simulink model "dynamic_resistance_charging"  (R2023a)
settings: Solver=VariableStepAuto  StartTime=0.0  StopTime=300  FixedStep=5e-6  RelTol=1e-3
undefined symbols (not defined in the file): Ion, Lithium
libraries: spsSeriesRLCBranchLib x8, spsMosfetLib x5, spsCurrentMeasurementLib x4, spsBatteryLib x3, spsDCVoltageSourceLib x1, spsGroundLib x1, sps_lib x1
settings Model: SimulationMode=accelerator  Creator=91620  LastModifiedBy=91620

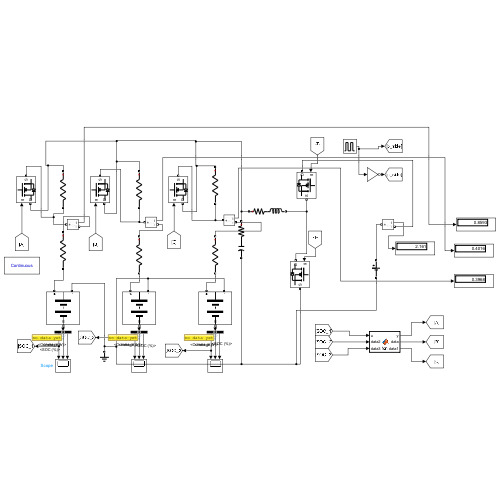
[thumbnail: Simulink's stored preview of the top-level diagram]
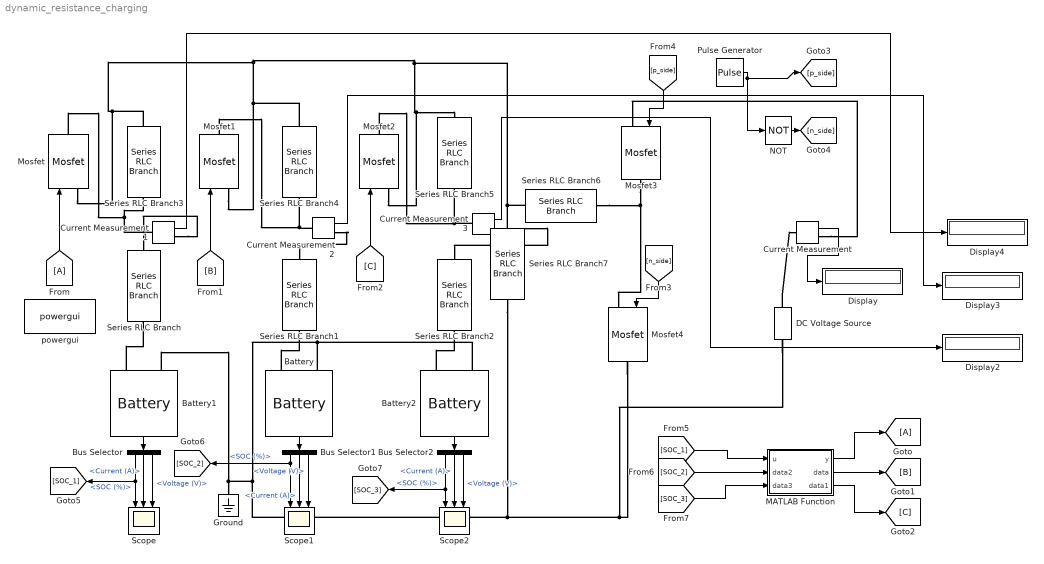
== system dynamic_resistance_charging ==
  Battery : spsBatteryLib/Battery  BatType=Lithium-Ion  ShowTempParam=off  ThermalPreset=no  ShowAgeParam=off  NomV=27  NomQ=5.4  SOC=40  Batt_Tr=1  PresetModel=on  MaxQ=5.4  MinV=20.25  FullV=31.4277  Dis_rate=2.3478  R=0.05  Normal_OP=4.8835  expZone="[29.1704     0.265304]"  current=[6.5 13 32.5]  Units=Time  Tci=20  NomT=20  T2=-30  MaxQ2=4.8  FullV2=7.1  Normal_OP2=5.655  expZone2="[6.58           1]"  Rca=0.6  ti=2000  Dp=0  Neq0=0  Tsim=1e6  Ta1=25  Qeol=5.4*0.9  Reol=0.013333*1.2  Char_age=[2.3478, 3]  Dis_age=[2.3478, 10]  N1=1500  N2=10500  N3=1000  N4=1400  Ta2=45  N5=950
  Battery1 : spsBatteryLib/Battery  BatType=Lithium-Ion  ShowTempParam=off  ThermalPreset=no  ShowAgeParam=off  NomV=27  NomQ=5.4  SOC=20  Batt_Tr=1  PresetModel=on  MaxQ=5.4  MinV=20.25  FullV=31.4277  Dis_rate=2.3478  R=0.05  Normal_OP=4.8835  expZone="[29.1704     0.265304]"  current=[6.5 13 32.5]  Units=Time  Tci=20  NomT=20  T2=-30  MaxQ2=4.8  FullV2=7.1  Normal_OP2=5.655  expZone2="[6.58           1]"  Rca=0.6  ti=2000  Dp=0  Neq0=0  Tsim=1e6  Ta1=25  Qeol=5.4*0.9  Reol=0.013333*1.2  Char_age=[2.3478, 3]  Dis_age=[2.3478, 10]  N1=1500  N2=10500  N3=1000  N4=1400  Ta2=45  N5=950
  Battery2 : spsBatteryLib/Battery  BatType=Lithium-Ion  ShowTempParam=off  ThermalPreset=no  ShowAgeParam=off  NomV=27  NomQ=5.4  SOC=42  Batt_Tr=1  PresetModel=on  MaxQ=5.4  MinV=20.25  FullV=31.4277  Dis_rate=2.3478  R=0.05  Normal_OP=4.8835  expZone="[29.1704     0.265304]"  current=[6.5 13 32.5]  Units=Time  Tci=20  NomT=20  T2=-30  MaxQ2=4.8  FullV2=7.1  Normal_OP2=5.655  expZone2="[6.58           1]"  Rca=0.6  ti=2000  Dp=0  Neq0=0  Tsim=1e6  Ta1=25  Qeol=5.4*0.9  Reol=0.013333*1.2  Char_age=[2.3478, 3]  Dis_age=[2.3478, 10]  N1=1500  N2=10500  N3=1000  N4=1400  Ta2=45  N5=950
  Bus Selector : BusSelector  OutputSignals=SOC (%),Current (A),Voltage (V)
  Bus Selector1 : BusSelector  OutputSignals=SOC (%),Current (A),Voltage (V)
  Bus Selector2 : BusSelector  OutputSignals=SOC (%),Current (A),Voltage (V)
  Current Measurement{,1..3} (4 alike) : spsCurrentMeasurementLib/Current Measurement  PhasorSimulation=off  OutputType=Complex  PSBequivalent=0
  DC Voltage Source : spsDCVoltageSourceLib/DC Voltage Source  Amplitude=48  Measurements=None
  Display{,2..4} (4 alike) : Display
  From : From
  Goto : Goto
  Ground : spsGroundLib/Ground  LConnTagsString=a
  MATLAB Function : MATLAB Function  TreatAsAtomicUnit=on
  Mosfet{,1..4} (5 alike) : spsMosfetLib/Mosfet  Ron=0.1  Lon=0  Rd=0.01  Vfd=0  IC=0  Rs=1e5  Cs=inf  Measurements=off
  NOT : Logic  Operator=NOT  IconShape=distinctive  AllPortsSameDT=off  OutDataTypeStr=boolean
  Pulse Generator : DiscretePulseGenerator  PulseType=Time based  Period=1e-4  PulseWidth=70
  Scope : Scope  NumInputPorts=3
  Scope1 : Scope  NumInputPorts=3
  Scope2 : Scope  NumInputPorts=3
  Series RLC Branch : spsSeriesRLCBranchLib/Series RLC Branch  LConnTagsString=__new0  RConnTagsString=__new0  BranchType=R  Resistance=0.54  Inductance=1e-3  SetiL0=off  InitialCurrent=0  Capacitance=1e-6  Setx0=off  InitialVoltage=0  Measurements=None
  Series RLC Branch1 : spsSeriesRLCBranchLib/Series RLC Branch  LConnTagsString=__new0  RConnTagsString=__new0  BranchType=R  Resistance=0.54  Inductance=1e-3  SetiL0=off  InitialCurrent=0  Capacitance=1e-6  Setx0=off  InitialVoltage=0  Measurements=None
  Series RLC Branch2 : spsSeriesRLCBranchLib/Series RLC Branch  LConnTagsString=__new0  RConnTagsString=__new0  BranchType=R  Resistance=0.54  Inductance=1e-3  SetiL0=off  InitialCurrent=0  Capacitance=1e-6  Setx0=off  InitialVoltage=0  Measurements=None
  Series RLC Branch3 : spsSeriesRLCBranchLib/Series RLC Branch  LConnTagsString=__new0  RConnTagsString=__new0  BranchType=R  Resistance=5.4  Inductance=1e-3  SetiL0=off  InitialCurrent=0  Capacitance=1e-6  Setx0=off  InitialVoltage=0  Measurements=None
  Series RLC Branch4 : spsSeriesRLCBranchLib/Series RLC Branch  LConnTagsString=__new0  RConnTagsString=__new0  BranchType=R  Resistance=5.4  Inductance=1e-3  SetiL0=off  InitialCurrent=0  Capacitance=1e-6  Setx0=off  InitialVoltage=0  Measurements=None
  Series RLC Branch5 : spsSeriesRLCBranchLib/Series RLC Branch  LConnTagsString=__new0  RConnTagsString=__new0  BranchType=R  Resistance=5.4  Inductance=1e-3  SetiL0=off  InitialCurrent=0  Capacitance=1e-6  Setx0=off  InitialVoltage=0  Measurements=None
  Series RLC Branch6 : spsSeriesRLCBranchLib/Series RLC Branch  LConnTagsString=__new0  RConnTagsString=__new0  BranchType=RL  Resistance=0.1  Inductance=1e-3  SetiL0=off  InitialCurrent=0  Capacitance=1e-6  Setx0=off  InitialVoltage=0  Measurements=None
  Series RLC Branch7 : spsSeriesRLCBranchLib/Series RLC Branch  LConnTagsString=__new0  RConnTagsString=__new0  BranchType=RC  Resistance=0.001  Inductance=1e-3  SetiL0=off  InitialCurrent=0  Capacitance=1000e-6  Setx0=off  InitialVoltage=0  Measurements=None
  powergui : sps_lib/powergui  Priority=1  SimulationMode=Continuous  SampleTime=5e-6  frequency=60  Iterations=50  frequencyindice=0  Pbase=100e6  ErrMax=1e-4  UnitsV=kV  UnitsW=MW  buscounter=0  FunctionMessages=off  echomessages=off  EnableUseOfTLC=off  CurrentSourceSwitches=off  DisableSnubberDevices=off  DisableRonSwitches=off  DisableVfSwitches=off  DisplayEquations=off  AutomaticDiscreteSolvers=off  SolverType=Tustin/Backward Euler (TBE)  Interpol=off  ExternalGateDelay=off  methode=off  Ts=100  x0status=blocks  SPID=on  SwTol=0  HookPort=off  NonlinearTolerance=1e-4  nMaxIteration=100  ContinueOnMaxIteration=off  RestoreLinks=warning  ResistiveCurrentMeasurement=off  Frange=[0:2:500]  Ylog=off  Xlog=on  ShowGrid=off  save=off  variable=ZData  structure=0  ZoomFFT=off  StartTime=0.0  cycles=1  DisplayStyle=1  fundamental=60  FreqAxis=off  MaxFrequency=1000  frequencyindicesteady=1  RmsSteady=1  display=off
  wires:
  [B] -> Mosfet1/1
  NOT/1 -> [n_side]
  Bus Selector/3 -> Scope/3  "<Voltage (V)>"
  MATLAB Function/2(data) -> [B]
  [SOC_2] -> MATLAB Function/2(data2)
  [SOC_1] -> MATLAB Function/1(u)
  Bus Selector2/1 -> [SOC_3], Scope2/1  "<SOC (%)>"
  Bus Selector/2 -> Scope/2  "<Current (A)>"
  Bus Selector2/3 -> Scope2/3  "<Voltage (V)>"
  Bus Selector2/2 -> Scope2/2  "<Current (A)>"
  MATLAB Function/1(y) -> Goto/1
  Bus Selector1/1 -> Scope1/1, [SOC_2]  "<SOC (%)>"
  Battery/1 -> Bus Selector1/1
  MATLAB Function/3(data1) -> [C]
  Bus Selector1/3 -> Scope1/3  "<Voltage (V)>"
  Pulse Generator/1 -> [p_side], NOT/1
  Bus Selector/1 -> [SOC_1], Scope/1  "<SOC (%)>"
  [n_side] -> Mosfet4/1
  Bus Selector1/2 -> Scope1/2  "<Current (A)>"
  Battery1/1 -> Bus Selector/1
  [C] -> Mosfet2/1
  From/1 -> Mosfet/1
  [SOC_3] -> MATLAB Function/3(data3)
  [p_side] -> Mosfet3/1
  Battery2/1 -> Bus Selector2/1
  Current Measurement/1 -> Display/1
  Current Measurement1/1 -> Display4/1
  Current Measurement2/1 -> Display3/1
  Current Measurement3/1 -> Display2/1
  connections:
  Mosfet4/RConn1 -- DC Voltage Source/LConn1 -- Series RLC Branch7/RConn1 -- Battery2/LConn2 -- Battery/LConn2 -- Battery1/LConn2 -- Ground/LConn1
  Mosfet3/RConn1 -- Series RLC Branch6/RConn1 -- Mosfet4/LConn1
  Current Measurement3/LConn1 -- Mosfet2/RConn1 -- Series RLC Branch5/RConn1
  Current Measurement1/LConn1 -- Mosfet/RConn1 -- Series RLC Branch3/RConn1
  Current Measurement2/LConn1 -- Mosfet1/RConn1 -- Series RLC Branch4/RConn1
  Battery1/LConn1 -- Series RLC Branch/RConn1
  Battery2/LConn1 -- Series RLC Branch2/RConn1
  Battery/LConn1 -- Series RLC Branch1/RConn1
  DC Voltage Source/RConn1 -- Current Measurement/LConn1
  Current Measurement/RConn1 -- Mosfet3/LConn1
  Current Measurement1/RConn1 -- Series RLC Branch/LConn1
  Current Measurement2/RConn1 -- Series RLC Branch1/LConn1
  Current Measurement3/RConn1 -- Series RLC Branch2/LConn1
  Series RLC Branch3/LConn1 -- Mosfet/LConn1 -- Mosfet1/LConn1 -- Series RLC Branch4/LConn1 -- Series RLC Branch6/LConn1 -- Series RLC Branch7/LConn1 -- Mosfet2/LConn1 -- Series RLC Branch5/LConn1

== matlab function dynamic_resistance_charging/MATLAB Function ==
  data: u input; y output; data output; data1 output; data2 input; data3 input
function [y,data, data1] = fcn(u, data2, data3)
maxi = -1;
if(data2> maxi)
    maxi = data2;
end
if(data3 > maxi)
    maxi = data3;
end
if(u > maxi)
    maxi = u;
end

y= 1;
    data=1;
    data1=1;
if((u+60) > 99)
    y= 0;
end
if((data2+60) > 99)
    data= 0;
end
if((data3+60) > 99)
    data1= 0;
end
;


%SOC_1->u
%SOC_2->data2
%SOC_3->data3

%A->y
%B->data
%C->data1
